simulink model "montajeLQR"  (R2021a)
settings: Solver=VariableStepAuto  StartTime=0.0  StopTime=20  RelTol=1e-3
undefined symbols (not defined in the file): k
settings Model: Creator=jjres  LastModifiedBy=jjres

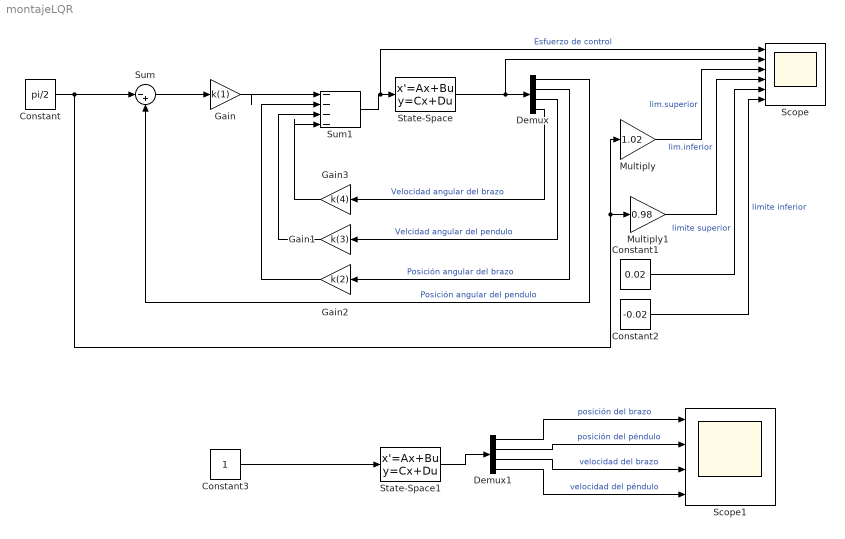
== system montajeLQR ==
  Constant : Constant  Value=pi/2
  Constant1 : Constant  Value=0.02
  Constant2 : Constant  Value=-0.02
  Constant3 : Constant
  Demux : Demux
  Demux1 : Demux
  Gain : Gain  Gain=k(1)
  Gain1 : Gain  Gain=k(3)
  Gain2 : Gain  Gain=k(2)
  Gain3 : Gain  Gain=k(4)
  Multiply : Gain  Gain=1.02
  Multiply1 : Gain  Gain=0.98
  Scope : Scope  NumInputPorts=6
  Scope1 : Scope  NumInputPorts=4
  State-Space : StateSpace  A=[0 0 1 0 ; 0 0 0 1; 0 -28.1714 -3.21283 0.928499; 0 86.1096 -3.17547 -2.83808]  B=[0; 0 ; 9.39423 ; 9.28499]  C=[1 0 0 0; 0 1 0 0; 0 0 1 0; 0 0 0 1]  D=[0;0;0;0]  InitialCondition=0
  State-Space1 : StateSpace  A=[0 0 1 0 ; 0 0 0 1; 0 -28.1714 -3.21283 0.928499; 0 86.1096 -3.17547 -2.83808]  B=[0; 0 ; 9.39423 ; 9.28499]  C=[1 0 0 0; 0 1 0 0; 0 0 1 0; 0 0 0 1]  D=[0;0;0;0]  InitialCondition=0
  Sum : Sum  Inputs=|-+
  Sum1 : Sum  Inputs=|----
  wires:
  Gain/1 -> Sum1/1
  Sum/1 -> Gain/1
  Constant/1 -> Multiply1/1, Multiply/1, Sum/1
  Sum1/1 -> Scope/1, State-Space/1  "Esfuerzo de control"
  State-Space/1 -> Scope/2, Demux/1
  Demux/2 -> Gain2/1  "Posición angular del brazo"
  Demux/1 -> Sum/2  "Posición angular del pendulo"
  Demux/3 -> Gain1/1  "Velcidad angular del pendulo"
  Demux/4 -> Gain3/1  "Velocidad angular del brazo"
  Multiply/1 -> Scope/3  "lim.superior"
  Multiply1/1 -> Scope/4  "lim.inferior"
  Constant1/1 -> Scope/5  "limite superior"
  Constant2/1 -> Scope/6  "limite inferior"
  Gain3/1 -> Sum1/4
  Gain1/1 -> Sum1/3
  Gain2/1 -> Sum1/2
  Constant3/1 -> State-Space1/1
  State-Space1/1 -> Demux1/1
  Demux1/1 -> Scope1/1  "posición del brazo"
  Demux1/2 -> Scope1/2  "posición del péndulo"
  Demux1/3 -> Scope1/3  "velocidad del brazo"
  Demux1/4 -> Scope1/4  "velocidad del péndulo"
